simulink model "SiL_gram"  (R2025b)
settings: Solver=ode2  StartTime=0.0  StopTime=t_end  FixedStep=1/400  RelTol=1e-3
PreLoadFcn:
  | stepsize_sim = evalin('base', get_param(bdroot, 'FixedStep'));
undefined symbols (not defined in the file or in its folder): defaultConsts, defaultWP, DiscIntNeverNeededParam, dspblkCoreblockFVToolHelper, gcbh, navConsts, sensors, stepsize_ctrl
libraries: simulink x7, sharedutil x1, sharedtransform x1, aerolibanimutils x1
(part 2 of 3)

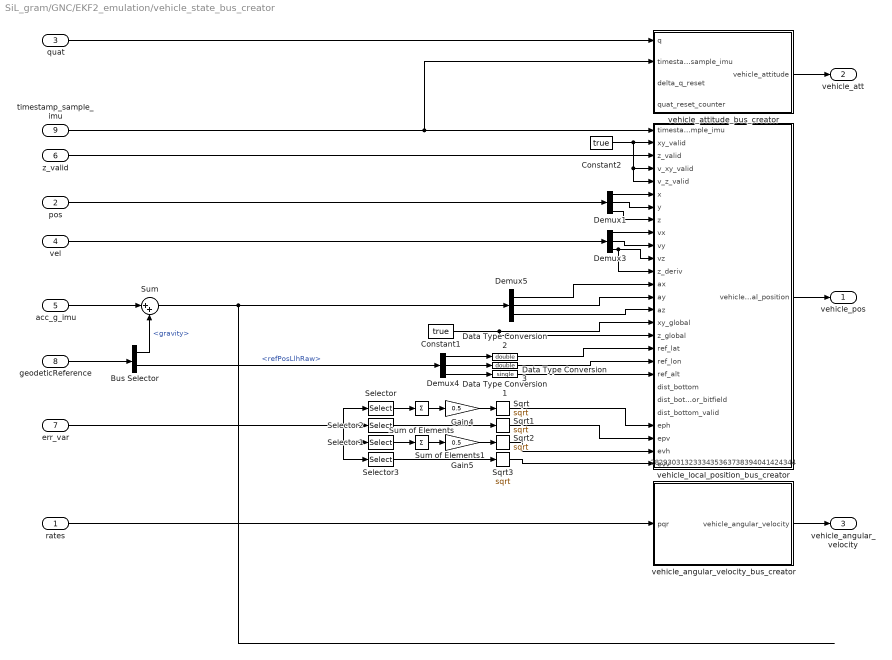
== system SiL_gram/GNC/EKF2_emulation/vehicle_state_bus_creator ==
  rates : Inport
  pos : Inport  Port=2  OutDataTypeStr=single  PortDimensions=3
  quat : Inport  Port=3
  vel : Inport  Port=4
  acc_g_imu : Inport  Port=5
  z_valid : Inport  Port=6  OutDataTypeStr=boolean
  err_var : Inport  Port=7
  geodeticReference : Inport  Port=8  OutDataTypeStr=Bus: ifr_geodeticReference
  timestamp_sample_imu : Inport  Port=9
  Bus Selector : BusSelector  OutputSignals=gravity,refPosLlhRaw
  Constant1 : Constant  Value=true  OutDataTypeStr=boolean
  Constant2 : Constant  Value=true  OutDataTypeStr=boolean
  Data Type Conversion1 : DataTypeConversion  OutDataTypeStr=double  SaturateOnIntegerOverflow=off  RndMeth=Floor
  Data Type Conversion2 : DataTypeConversion  OutDataTypeStr=double  SaturateOnIntegerOverflow=off  RndMeth=Floor
  Data Type Conversion3 : DataTypeConversion  OutDataTypeStr=single  SaturateOnIntegerOverflow=off  RndMeth=Floor
  Demux{1,3..5} (4 alike) : Demux  Outputs=3
  Gain4 : Gain  Gain=0.5  OutDataTypeStr=single
  Gain5 : Gain  Gain=0.5  OutDataTypeStr=single
  Selector : Selector  InputPortWidth=9  IndexOptions=Index vector (dialog)  Indices=[1 2]  OutputSizes=1
  Selector1 : Selector  InputPortWidth=9  IndexOptions=Index vector (dialog)  Indices=[4 5]  OutputSizes=1
  Selector2 : Selector  InputPortWidth=9  IndexOptions=Index vector (dialog)  Indices=3  OutputSizes=1
  Selector3 : Selector  InputPortWidth=9  IndexOptions=Index vector (dialog)  Indices=6  OutputSizes=1
  Sqrt{,1..3} (4 alike) : Sqrt
  Sum : Sum  Inputs=|++
  Sum of Elements : Sum  Inputs=+
  Sum of Elements1 : Sum  Inputs=+
  vehicle_angular_velocity_bus_creator : Subsystem
  vehicle_attitude_bus_creator : Subsystem
  vehicle_local_position_bus_creator : Subsystem
      settings: PortSchema="{\"entries\":[{\"content\":{\"sides\":[{\"content\":{\"connectorIds\":[\"In1\",\"In2\",\"In3\",\"In4\",\"In5\",\"In6\",\"In7\",\"In8\",\"In9\",\"In10\",\"In11\",\"In12\",\"In13\",\"In14\",\"In15\",\"In16\",\"In17\",\"In18\",\"In19\",\"In20\",\"In21\",\"In22\",\"In23\",\"In24\",\"In25\",\"In26\",\"In27\"]},\"type\":\"ConnectorPlacement.EquallySpacedRectSide\",\"uuid\":\"d7b85d5c-5599-4e88-82f1-b7fab1ef21b9\"},{\"content\":{\"connectorIds\":[\"Out1\"],\"side\":\"RIGHT\"},\"type\":\"ConnectorPlacement.EquallySpacedRectSide\",\"uuid\":\"699d4796-c4a5-400d-ae7f-d0fe809a1d5f\"},{\"content\":{\"side\":\"TOP\"},\"type\":\"ConnectorPlacement.EquallySpacedRectSide\",\"uuid\":\"a5a49804-595b-4b61-9074-ba74b998a229\"},{\"content\":{\"connectorIds\":[\"In28\",\"In29\",\"In30\",\"In31\",\"In32\",\"In33\",\"In34\",\"In35\",\"In36\",\"In37\",\"In38\",\"In39\",\"In40\",\"In41\",\"In42\",\"In43\",\"In44\"],\"side\":\"BOTTOM\"},\"type\":\"ConnectorPlacement.EquallySpacedRectSide\",\"uuid\":\"117ce955-faca-4d28-9193-e1fd103a05b2\"}]},\"type\":\"ConnectorPlacement.EquallySpacedConnector\",\"uuid\":\"4d71e442-d8d4-4e8b-a7eb-573f45a4a9ae\"}],\"packageUris\":[\"http://schema.mathworks.com/mf0/Connector/R2020b\"],\"version\":\"1.0\"}"
  vehicle_pos : Outport  OutDataTypeStr=Bus: vehicle_local_position_bus  VectorParamsAs1DForOutWhenUnconnected=off
  vehicle_att : Outport  Port=2  OutDataTypeStr=Bus: vehicle_attitude_bus  VectorParamsAs1DForOutWhenUnconnected=off
  vehicle_angular_velocity : Outport  Port=3  OutDataTypeStr=Bus: vehicle_angular_velocity_bus
  wires:
  rates/1 -> vehicle_angular_velocity_bus_creator/1(pqr)
  z_valid/1 -> vehicle_local_position_bus_creator/3(z_valid)
  Constant2/1 -> vehicle_local_position_bus_creator/4(v_xy_valid), vehicle_local_position_bus_creator/5(v_z_valid), vehicle_local_position_bus_creator/2(xy_valid)
  Demux5/3 -> vehicle_local_position_bus_creator/15(az)
  Data Type Conversion1/1 -> vehicle_local_position_bus_creator/19(ref_lon)
  Sqrt3/1 -> vehicle_local_position_bus_creator/27(evv)
  Sqrt2/1 -> vehicle_local_position_bus_creator/26(evh)
  vel/1 -> Demux3/1
  Demux4/3 -> Data Type Conversion3/1
  Sqrt1/1 -> vehicle_local_position_bus_creator/25(epv)
  Demux1/3 -> vehicle_local_position_bus_creator/8(z)
  Demux1/2 -> vehicle_local_position_bus_creator/7(y)
  Demux5/2 -> vehicle_local_position_bus_creator/14(ay)
  Constant1/1 -> vehicle_local_position_bus_creator/17(z_global), vehicle_local_position_bus_creator/16(xy_global)
  Demux1/1 -> vehicle_local_position_bus_creator/6(x)
  Data Type Conversion2/1 -> vehicle_local_position_bus_creator/18(ref_lat)
  Sqrt/1 -> vehicle_local_position_bus_creator/24(eph)
  Data Type Conversion3/1 -> vehicle_local_position_bus_creator/20(ref_alt)
  Demux3/3 -> vehicle_local_position_bus_creator/12(z_deriv), vehicle_local_position_bus_creator/11(vz)
  pos/1 -> Demux1/1
  Demux5/1 -> vehicle_local_position_bus_creator/13(ax)
  Demux3/1 -> vehicle_local_position_bus_creator/9(vx)
  Demux3/2 -> vehicle_local_position_bus_creator/10(vy)
  Selector1/1 -> Sum of Elements1/1
  Selector/1 -> Sum of Elements/1
  Selector3/1 -> Sqrt3/1
  Sum of Elements1/1 -> Gain5/1
  Sum of Elements/1 -> Gain4/1
  Selector2/1 -> Sqrt1/1
  err_var/1 -> Selector/1, Selector1/1, Selector3/1, Selector2/1
  Gain5/1 -> Sqrt2/1
  Gain4/1 -> Sqrt/1
  Sum/1 -> Demux5/1
  Bus Selector/2 -> Demux4/1  "<refPosLlhRaw>"
  Bus Selector/1 -> Sum/2  "<gravity>"
  geodeticReference/1 -> Bus Selector/1
  acc_g_imu/1 -> Sum/1
  quat/1 -> vehicle_attitude_bus_creator/1(q)
  timestamp_sample_imu/1 -> vehicle_attitude_bus_creator/2(timestamp_sample_imu), vehicle_local_position_bus_creator/1(timestamp_sample_imu)
  Demux4/2 -> Data Type Conversion1/1
  Demux4/1 -> Data Type Conversion2/1
  vehicle_local_position_bus_creator/1(vehicle_local_position) -> vehicle_pos/1
  vehicle_attitude_bus_creator/1(vehicle_attitude) -> vehicle_att/1
  vehicle_angular_velocity_bus_creator/1(vehicle_angular_velocity) -> vehicle_angular_velocity/1

== system SiL_gram/GNC/mavlink_receiver.cpp/  ==
  note: integration_timespan
      | ground_distance_m
  air : Inport  OutDataTypeStr=Bus: ifr_airdata
  Bus Creator1 : BusCreator  Inputs=21  OutDataTypeStr=Bus: optical_flow_bus
      settings: InheritFromInputs=off
  Bus Selector : BusSelector  OutputSignals=isValid,alpha_volt,beta_volt
  Constant1 : Constant  Value=zeros(3,1)
  Constant2 : Constant  Value=0  OutDataTypeStr=uint8
  Constant3 : Constant  Value=0  OutDataTypeStr=uint8
  Constant4 : Constant  Value=zeros(7,1)
  Constant5 : Constant  Value=0  OutDataTypeStr=single
  Constant6 : Constant  OutDataTypeStr=uint32
  Data Type Conversion{1..3,8..12} (8 alike) : DataTypeConversion  OutDataTypeStr=single  SaturateOnIntegerOverflow=off  RndMeth=Floor
  Data Type Conversion4 : DataTypeConversion  OutDataTypeStr=uint32  SaturateOnIntegerOverflow=off  RndMeth=Floor
  Data Type Conversion5 : DataTypeConversion  OutDataTypeStr=uint16  SaturateOnIntegerOverflow=off  RndMeth=Floor
  Data Type Conversion6 : DataTypeConversion  OutDataTypeStr=int16  SaturateOnIntegerOverflow=off  RndMeth=Floor
  Data Type Conversion7 : DataTypeConversion  OutDataTypeStr=uint8  SaturateOnIntegerOverflow=off  RndMeth=Floor
  Demux : Demux  Outputs=7
  Demux1 : Demux  Outputs=3
  opFlow : Outport  OutDataTypeStr=Bus: optical_flow_bus
  wires:
  Data Type Conversion8/1 -> Bus Creator1/14
  Constant1/1 -> Demux1/1
  Data Type Conversion2/1 -> Bus Creator1/6
  Data Type Conversion6/1 -> Bus Creator1/12
  Demux1/3 -> Data Type Conversion3/1
  Data Type Conversion3/1 -> Bus Creator1/7
  Demux/7 -> Data Type Conversion11/1
  Constant4/1 -> Demux/1
  Demux/4 -> Data Type Conversion7/1
  Data Type Conversion4/1 -> Bus Creator1/10
  Demux/5 -> Data Type Conversion8/1
  Demux/2 -> Data Type Conversion5/1
  Demux1/1 -> Data Type Conversion1/1
  Demux/6 -> Data Type Conversion9/1
  Constant5/1 -> Bus Creator1/8  "ground_distance_m"
  Bus Creator1/1 -> opFlow/1
  Constant3/1 -> Bus Creator1/2
  Data Type Conversion7/1 -> Bus Creator1/13
  Constant6/1 -> Bus Creator1/9  "integration_timespan"
  Data Type Conversion5/1 -> Bus Creator1/11
  Demux1/2 -> Data Type Conversion2/1
  Data Type Conversion11/1 -> Bus Creator1/16
  Demux/3 -> Data Type Conversion6/1
  Data Type Conversion9/1 -> Bus Creator1/15
  Data Type Conversion1/1 -> Bus Creator1/5
  Demux/1 -> Data Type Conversion4/1
  Data Type Conversion12/1 -> Bus Creator1/3
  air/1 -> Bus Selector/1
  Bus Selector/1 -> Bus Creator1/1  "<isValid>"
  Data Type Conversion10/1 -> Bus Creator1/4
  Bus Selector/3 -> Data Type Conversion10/1  "<beta_volt>"
  Bus Selector/2 -> Data Type Conversion12/1  "<alpha_volt>"
  Constant2/1 -> Bus Creator1/21, Bus Creator1/20, Bus Creator1/19, Bus Creator1/18, Bus Creator1/17

== system SiL_gram/GNC/mavlink_receiver.cpp/   ==
  Lidar : Inport  OutDataTypeStr=Bus: ifr_lidar
  Bus Creator1 : BusCreator  Inputs=31  OutDataTypeStr=Bus: distance_sensor_bus
      settings: InheritFromInputs=off
  Bus Selector : BusSelector  OutputSignals=isValid,distance
  Constant : Constant  Value=navConsts.lidarMinRange  OutDataTypeStr=single
  Constant1 : Constant  Value=navConsts.lidarMaxRange  OutDataTypeStr=single
  Constant11 : Constant  Value=zeros(4,1)  OutDataTypeStr=single
  Constant2 : Constant  Value=0  OutDataTypeStr=uint8
  Constant3 : Constant  OutDataTypeStr=uint8
  Constant4 : Constant  Value=0  OutDataTypeStr=int8
  Constant5 : Constant  OutDataTypeStr=uint8
  Constant6 : Constant  OutDataTypeStr=uint32
  Constant7 : Constant  Value=0  OutDataTypeStr=single
  Constant8 : Constant  Value=0  OutDataTypeStr=single
  Constant9 : Constant  Value=0  OutDataTypeStr=single
  lidar : Outport  OutDataTypeStr=Bus: distance_sensor_bus
  wires:
  Bus Creator1/1 -> lidar/1
  Lidar/1 -> Bus Selector/1
  Constant5/1 -> Bus Creator1/9  "MAV_DISTANCE_SENSOR_LASER"
  Constant/1 -> Bus Creator1/3
  Constant1/1 -> Bus Creator1/4
  Bus Selector/1 -> Bus Creator1/1  "<isValid>"
  Constant7/1 -> Bus Creator1/6
  Constant3/1 -> Bus Creator1/17  "ROTATION_DOWNWARD_FACING"
  Bus Selector/2 -> Bus Creator1/5  "<distance>"
  Constant4/1 -> Bus Creator1/7
  Constant6/1 -> Bus Creator1/2
  Constant8/1 -> Bus Creator1/13
  Constant9/1 -> Bus Creator1/14
  Constant11/1 -> Bus Creator1/15
  Constant2/1 -> Bus Creator1/12, Bus Creator1/11, Bus Creator1/10, Bus Creator1/8, Bus Creator1/31, Bus Creator1/30, Bus Creator1/29, Bus Creator1/28, Bus Creator1/27, Bus Creator1/26, Bus Creator1/25, Bus Creator1/24, Bus Creator1/23, Bus Creator1/22, Bus Creator1/21, Bus Creator1/20, Bus Creator1/19, Bus Creator1/18, Bus Creator1/16

== system SiL_gram/GNC/mavlink_receiver.cpp/    ==
  air : Inport  OutDataTypeStr=Bus: ifr_airdata
  Bus Creator1 : BusCreator  Inputs=6  OutDataTypeStr=Bus: airspeed_bus
      settings: InheritFromInputs=off
  Bus Selector : BusSelector  OutputSignals=isValid,V_a
  Cast To Double : DataTypeConversion  OutDataTypeStr=double  SaturateOnIntegerOverflow=off  RndMeth=Floor
  Constant1 : Constant  Value=0  OutDataTypeStr=single
  Constant2 : Constant  Value=0  OutDataTypeStr=single
  Constant3 : Constant  Value=0  OutDataTypeStr=single
  Data Type Conversion : DataTypeConversion  OutDataTypeStr=single  SaturateOnIntegerOverflow=off  RndMeth=Floor
  airdata : Outport  OutDataTypeStr=Bus: airspeed_bus
  wires:
  air/1 -> Bus Selector/1
  Data Type Conversion/1 -> Bus Creator1/3  "indicated_airspeed_m_s"
  Constant3/1 -> Bus Creator1/5  "air_temperature_celsius"
  Constant2/1 -> Bus Creator1/6  "confidence"
  Constant1/1 -> Bus Creator1/4  "true_airspeed_m_s"
  Bus Selector/1 -> Cast To Double/1, Bus Creator1/1  "<isValid>"
  Bus Creator1/1 -> airdata/1
  Bus Selector/2 -> Data Type Conversion/1  "<V_a>"
  Cast To Double/1 -> Bus Creator1/2  "true_airspeed_m_s"

== system SiL_gram/GNC/mavlink_receiver.cpp/ 1 ==
  air : Inport  OutDataTypeStr=Bus: ifr_airdata
  Bus Creator1 : BusCreator  Inputs=7  OutDataTypeStr=Bus: adc_report_bus
      settings: InheritFromInputs=off
  Bus Selector : BusSelector  OutputSignals=isValid,beta_volt,alpha_volt
  Constant : Constant  Value=[0,1,2,3,4,8,10,11,12,13,14,16]  OutDataTypeStr=int16
  Constant1 : Constant  Value=zeros(4,1)  OutDataTypeStr=single
  Constant2 : Constant  Value=zeros(5,1)  OutDataTypeStr=single
  Constant3 : Constant  Value=0  OutDataTypeStr=single
  Constant4 : Constant  OutDataTypeStr=uint32
  Constant5 : Constant  Value=zeros(12,1)  OutDataTypeStr=int32
  Constant6 : Constant  Value=0  OutDataTypeStr=uint32
  Constant7 : Constant  Value=0  OutDataTypeStr=single
  Mux : Mux  Inputs=5
  adcReport : Outport  OutDataTypeStr=Bus: adc_report_bus
  wires:
  Bus Selector/3 -> Mux/4  "<alpha_volt>"
  Bus Selector/2 -> Mux/2  "<beta_volt>"
  Bus Selector/1 -> Bus Creator1/1  "<isValid>"
  air/1 -> Bus Selector/1
  Bus Creator1/1 -> adcReport/1
  Constant/1 -> Bus Creator1/3
  Mux/1 -> Bus Creator1/4
  Constant1/1 -> Mux/1
  Constant2/1 -> Mux/3
  Constant3/1 -> Mux/5
  Constant4/1 -> Bus Creator1/2
  Constant5/1 -> Bus Creator1/5
  Constant6/1 -> Bus Creator1/6
  Constant7/1 -> Bus Creator1/7

== system SiL_gram/GNC/mavlink_receiver.cpp/Arming ==
  Bus Creator : BusCreator  Inputs=9  OutDataTypeStr=Bus: actuator_armed_bus
      settings: InheritFromInputs=off
  armed : Constant  OutDataTypeStr=boolean
  force_failsafe : Constant  Value=0  OutDataTypeStr=boolean
  in_esc_calibration_mode : Constant  Value=0  OutDataTypeStr=boolean
  is_valid : Constant  Value=0  OutDataTypeStr=boolean
  lockdown : Constant  Value=0  OutDataTypeStr=boolean
  manual_lockdown : Constant  OutDataTypeStr=boolean
  prearmed : Constant  Value=0  OutDataTypeStr=boolean
  ready_to_arm : Constant  Value=0  OutDataTypeStr=boolean
  soft_stop : Constant  Value=0  OutDataTypeStr=boolean
  Armed : Outport  OutDataTypeStr=Bus: actuator_armed_bus
  wires:
  Bus Creator/1 -> Armed/1
  soft_stop/1 -> Bus Creator/9
  in_esc_calibration_mode/1 -> Bus Creator/8
  ready_to_arm/1 -> Bus Creator/4
  is_valid/1 -> Bus Creator/1
  lockdown/1 -> Bus Creator/5
  manual_lockdown/1 -> Bus Creator/6
  armed/1 -> Bus Creator/2  "armed"
  prearmed/1 -> Bus Creator/3
  force_failsafe/1 -> Bus Creator/7

== system SiL_gram/GNC/mavlink_receiver.cpp/Baro ==
  note: [Pa]
  p_alt : Inport
  Bus Creator1 : BusCreator  Inputs=7  OutDataTypeStr=Bus: sensor_baro_bus
      settings: InheritFromInputs=off
  Bus Selector : BusSelector  OutputSignals=isValid,height
  Cast To Double : DataTypeConversion  OutDataTypeStr=double  SaturateOnIntegerOverflow=off  RndMeth=Floor
  Constant1 : Constant  Value=0  OutDataTypeStr=uint32
  Constant2 : Constant  OutDataTypeStr=uint32
  Constant3 : Constant  Value=0  OutDataTypeStr=double
  Constant4 : Constant  Value=0  OutDataTypeStr=uint8
  Data Type Conversion1 : DataTypeConversion  OutDataTypeStr=single  SaturateOnIntegerOverflow=off  RndMeth=Floor
  Data Type Conversion10 : DataTypeConversion  OutDataTypeStr=single  SaturateOnIntegerOverflow=off  RndMeth=Floor
  height2baro : MATLAB Function  TreatAsAtomicUnit=on
  baro : Outport  OutDataTypeStr=Bus: sensor_baro_bus
  wires:
  Constant4/1 -> Bus Creator1/7  "error_count"
  Constant2/1 -> Bus Creator1/3  "device_id"
  Constant3/1 -> Data Type Conversion1/1  "error_count"
  height2baro/1(pressure) -> Data Type Conversion10/1
  Bus Creator1/1 -> baro/1
  Data Type Conversion1/1 -> Bus Creator1/5  "temp"
  Bus Selector/2 -> height2baro/1(height)  "<height>"
  Bus Selector/1 -> Cast To Double/1, Bus Creator1/1  "<isValid>"
  Constant1/1 -> Bus Creator1/6  "error_count"
  Data Type Conversion10/1 -> Bus Creator1/4  "pressure"
  p_alt/1 -> Bus Selector/1
  Cast To Double/1 -> Bus Creator1/2  "true_airspeed_m_s"

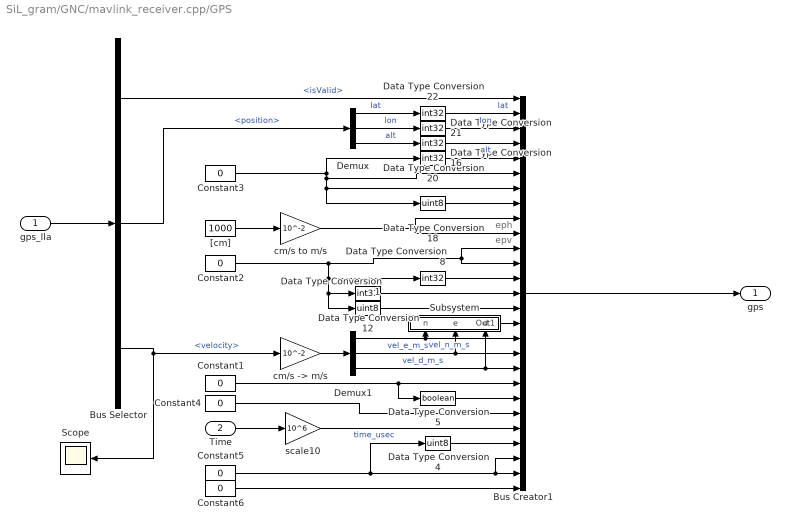
== system SiL_gram/GNC/mavlink_receiver.cpp/GPS ==
  note: eph
  note: epv
  gps_lla : Inport
  Time : Inport  Port=2
  Bus Creator1 : BusCreator  Inputs=27  OutDataTypeStr=Bus: vehicle_gps_position_bus
      settings: InheritFromInputs=off
  Bus Selector : BusSelector  OutputSignals=isValid,position,velocity
  Constant{1..3,5} (4 alike) : Constant  Value=0  OutDataTypeStr=single
  Constant4 : Constant  Value=0  OutDataTypeStr=int32
  Constant6 : Constant  Value=0  OutDataTypeStr=uint8
  Data Type Conversion1 : DataTypeConversion  OutDataTypeStr=uint8  SaturateOnIntegerOverflow=off  RndMeth=Floor
  Data Type Conversion{8,12,16,20..22} (6 alike) : DataTypeConversion  OutDataTypeStr=int32  SaturateOnIntegerOverflow=off  RndMeth=Floor
  Data Type Conversion18 : DataTypeConversion  OutDataTypeStr=uint8  SaturateOnIntegerOverflow=off  RndMeth=Floor
  Data Type Conversion4 : DataTypeConversion  OutDataTypeStr=uint8  SaturateOnIntegerOverflow=off  RndMeth=Floor
  Data Type Conversion5 : DataTypeConversion  OutDataTypeStr=boolean  SaturateOnIntegerOverflow=off  RndMeth=Floor
  Demux : Demux  Outputs=3
  Demux1 : Demux  Outputs=3
  Scope : Scope
      settings: ActiveDisplayYMinimum=-4879.31316  ActiveDisplayYMaximum=1977.92464
  Subsystem : Subsystem
      settings: PortSchema="{\"entries\":[{\"content\":{\"sides\":[{\"content\":{},\"type\":\"ConnectorPlacement.EquallySpacedRectSide\",\"uuid\":\"42608b9b-4e0b-4cd6-95a4-868653eebf85\"},{\"content\":{\"connectorIds\":[\"Out1\"],\"side\":\"RIGHT\"},\"type\":\"ConnectorPlacement.EquallySpacedRectSide\",\"uuid\":\"b8a148f6-1c9c-4225-91f9-202796ff464f\"},{\"content\":{\"side\":\"TOP\"},\"type\":\"ConnectorPlacement.EquallySpacedRectSide\",\"uuid\":\"0f80df07-b651-41b7-aa18-0093fc65c3ad\"},{\"content\":{\"connectorIds\":[\"In1\",\"In2\",\"In3\"],\"side\":\"BOTTOM\"},\"type\":\"ConnectorPlacement.EquallySpacedRectSide\",\"uuid\":\"f4234091-6e8c-4bc0-a362-f8928a822b26\"}]},\"type\":\"ConnectorPlacement.EquallySpacedConnector\",\"uuid\":\"4767cb59-0a97-4a99-80e8-760d373adfc4\"}],\"packageUris\":[\"http://schema.mathworks.com/mf0/Connector/R2020b\"],\"version\":\"1.0\"}"
  "[cm]" : Constant  Value=1000  OutDataTypeStr=single
  "cm/s -> m/s" : Gain  Gain=10^-2  OutDataTypeStr=single
  cm/s to m/s : Gain  Gain=10^-2  OutDataTypeStr=single
  scale10 : Gain  Gain=10^6  OutDataTypeStr=double
  gps : Outport  OutDataTypeStr=Bus: vehicle_gps_position_bus
  wires:
  Bus Selector/3 -> Scope/1, "cm/s -> m/s"/1  "<velocity>"
  Time/1 -> scale10/1
  Data Type Conversion22/1 -> Bus Creator1/2  "lat"
  Data Type Conversion21/1 -> Bus Creator1/3  "lon"
  Data Type Conversion20/1 -> Bus Creator1/4  "alt"
  Data Type Conversion18/1 -> Bus Creator1/8
  Data Type Conversion16/1 -> Bus Creator1/5
  Constant2/1 -> Bus Creator1/11, Bus Creator1/12, Data Type Conversion1/1, Data Type Conversion12/1, Data Type Conversion8/1
  Data Type Conversion12/1 -> Bus Creator1/14
  Data Type Conversion8/1 -> Bus Creator1/13
  Constant1/1 -> Bus Creator1/20, Data Type Conversion5/1
  Data Type Conversion5/1 -> Bus Creator1/21
  Data Type Conversion4/1 -> Bus Creator1/24
  Constant5/1 -> Data Type Conversion4/1, Bus Creator1/25, Bus Creator1/26
  scale10/1 -> Bus Creator1/23  "time_usec"
  Demux1/1 -> Subsystem/1(n), Bus Creator1/17  "vel_n_m_s"
  Demux1/2 -> Bus Creator1/18, Subsystem/2(e)  "vel_e_m_s"
  Demux1/3 -> Subsystem/3(d), Bus Creator1/19  "vel_d_m_s"
  Demux/3 -> Data Type Conversion20/1  "alt"
  Demux/2 -> Data Type Conversion21/1  "lon"
  Constant3/1 -> Data Type Conversion18/1, Bus Creator1/7, Bus Creator1/6, Data Type Conversion16/1
  Demux/1 -> Data Type Conversion22/1  "lat"
  Bus Creator1/1 -> gps/1
  Bus Selector/1 -> Bus Creator1/1  "<isValid>"
  gps_lla/1 -> Bus Selector/1
  Bus Selector/2 -> Demux/1  "<position>"
  "cm/s -> m/s"/1 -> Demux1/1
  "[cm]"/1 -> cm/s to m/s/1
  cm/s to m/s/1 -> Bus Creator1/9, Bus Creator1/10
  Constant4/1 -> Bus Creator1/22
  Data Type Conversion1/1 -> Bus Creator1/15
  Constant6/1 -> Bus Creator1/27
  Subsystem/1(Out1) -> Bus Creator1/16

== system SiL_gram/GNC/mavlink_receiver.cpp/InputRC ==
  note: 1 Thrust
      | 2 Aileron
      | 3 Elevator
      | 4 Rudder
      | 5 Tail surface right
      | 6 Tail surface left
      | 7 Mode switch
      | 8 Arming
      | 9 Safety
  note: [ Thrust ]
      | [ Aileron ]
      | [ Elevator ]
      | [ Rudder ]
      | [ NW ]
      | [ Mode ]
      | [ Safety ]
  note: Input from Gram RC:
      | 1 Thrust
      | 2 Aileron right
      | 3 Aileron left
      | 4 Flaperon right
      | 5 Flaperon left
      | 6 Elevator/Rudder right
      | 7 Elevator/Rudder left
      | 8 Gear
      | 9 Safety
      | 10 Arming
      | 11 Mode switch
      | 12 Elevator
      | 13 Rudder
  RC : Inport
  Bus Creator2 : BusCreator  Inputs=36  OutDataTypeStr=Bus: rc_channels_bus
      settings: InheritFromInputs=off
  Constant2 : Constant  Value=zeros(33,1)  OutDataTypeStr=uint8
  Constant3 : Constant  Value=zeros(12,1)  OutDataTypeStr=single
  Constant4 : Constant  Value=true
  Constant5 : Constant  Value=zeros(27,1)  OutDataTypeStr=int8
  Data Type Conversion : DataTypeConversion  OutDataTypeStr=single  SaturateOnIntegerOverflow=off  RndMeth=Floor
  Data Type Conversion1 : DataTypeConversion  OutDataTypeStr=double  SaturateOnIntegerOverflow=off  RndMeth=Floor
  Data Type Conversion2 : DataTypeConversion  OutDataTypeStr=boolean  SaturateOnIntegerOverflow=off  RndMeth=Floor
  Data Type Conversion4 : DataTypeConversion  OutDataTypeStr=uint8  SaturateOnIntegerOverflow=off  RndMeth=Floor
  Data Type Conversion6 : DataTypeConversion  OutDataTypeStr=single  SaturateOnIntegerOverflow=off  RndMeth=Floor
  Data Type Conversion7 : DataTypeConversion  OutDataTypeStr=uint8  SaturateOnIntegerOverflow=off  RndMeth=Floor
  Data Type Conversion8 : DataTypeConversion  OutDataTypeStr=uint32  SaturateOnIntegerOverflow=off  RndMeth=Floor
  Demux : Demux  Outputs=8
  Demux1 : Demux  Outputs=12
  Demux2 : Demux  Outputs=33
  Mux : Mux  Inputs=18
  Scope2 : Scope
      settings: ActiveDisplayYMinimum=-1.25  ActiveDisplayYMaximum=1.25
  Terminator1 : Terminator
  Terminator2 : Terminator
  rc_channels : Outport  OutDataTypeStr=Bus: rc_channels_bus
  wires:
  Demux/2 -> Mux/2
  Demux/6 -> Mux/7
  Demux/7 -> Mux/9
  Demux1/8 -> Mux/14
  Demux1/10 -> Mux/16
  Demux1/9 -> Mux/15
  RC/1 -> Data Type Conversion/1
  Data Type Conversion8/1 -> Bus Creator2/36
  Demux2/1 -> Bus Creator2/2
  Demux/5 -> Terminator1/1
  Demux1/11 -> Mux/17
  Data Type Conversion4/1 -> Bus Creator2/32
  Data Type Conversion1/1 -> Bus Creator2/30
  Demux2/32 -> Data Type Conversion2/1
  Demux2/29 -> Data Type Conversion1/1
  Demux2/9 -> Bus Creator2/10
  Constant5/1 -> Bus Creator2/33
  Demux2/26 -> Bus Creator2/27
  Demux2/17 -> Bus Creator2/18
  Demux2/10 -> Bus Creator2/11
  Data Type Conversion2/1 -> Bus Creator2/35
  Constant3/1 -> Demux1/1
  Demux2/31 -> Data Type Conversion7/1
  Constant2/1 -> Demux2/1
  Demux2/30 -> Data Type Conversion4/1
  Demux2/6 -> Bus Creator2/7
  Constant4/1 -> Bus Creator2/1
  Demux2/21 -> Bus Creator2/22
  Demux2/20 -> Bus Creator2/21
  Demux2/4 -> Bus Creator2/5
  Demux2/12 -> Bus Creator2/13
  Demux2/8 -> Bus Creator2/9
  Data Type Conversion6/1 -> Bus Creator2/31
  Demux2/22 -> Bus Creator2/23
  Demux1/12 -> Mux/18
  Demux2/23 -> Bus Creator2/24
  Demux2/24 -> Bus Creator2/25
  Demux2/19 -> Bus Creator2/20
  Demux2/13 -> Bus Creator2/14
  Demux2/2 -> Bus Creator2/3
  Mux/1 -> Data Type Conversion6/1, Scope2/1
  Demux2/33 -> Data Type Conversion8/1
  Demux2/11 -> Bus Creator2/12
  Demux2/3 -> Bus Creator2/4
  Demux2/25 -> Bus Creator2/26
  Demux2/16 -> Bus Creator2/17
  Demux2/7 -> Bus Creator2/8
  Demux2/14 -> Bus Creator2/15
  Data Type Conversion7/1 -> Bus Creator2/34
  Bus Creator2/1 -> rc_channels/1
  Demux2/15 -> Bus Creator2/16
  Demux/8 -> Terminator2/1
  Demux2/18 -> Bus Creator2/19
  Demux2/5 -> Bus Creator2/6
  Demux2/27 -> Bus Creator2/28
  Demux/1 -> Mux/1
  Demux1/6 -> Mux/12
  Data Type Conversion/1 -> Demux/1
  Demux2/28 -> Bus Creator2/29
  Demux1/2 -> Mux/6
  Demux/3 -> Mux/3
  Demux/4 -> Mux/4
  Demux1/7 -> Mux/13
  Demux1/1 -> Mux/5
  Demux1/3 -> Mux/8
  Demux1/4 -> Mux/10
  Demux1/5 -> Mux/11

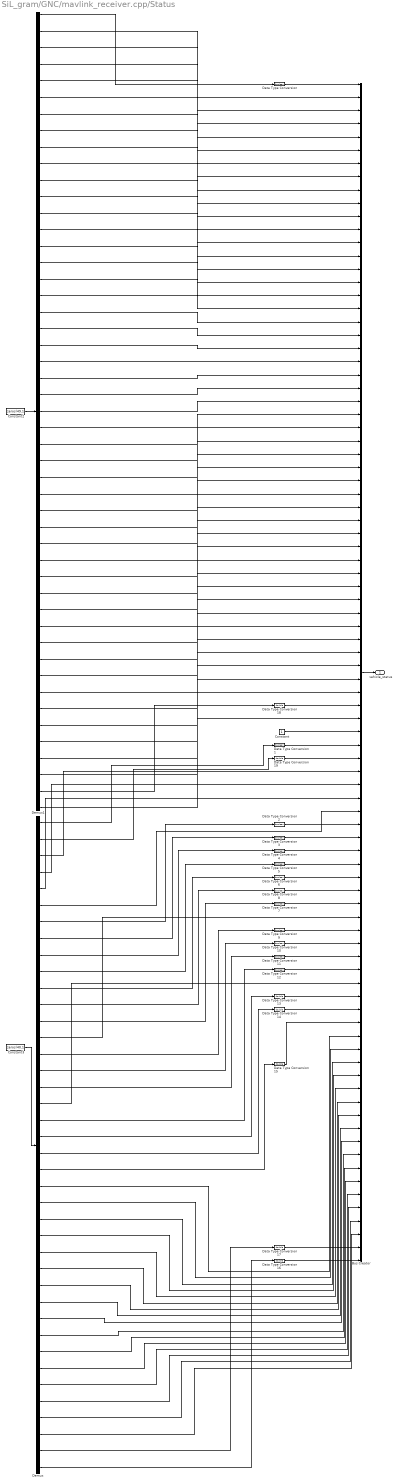
== system SiL_gram/GNC/mavlink_receiver.cpp/Status ==
  Bus Creator : BusCreator  Inputs=90  OutDataTypeStr=Bus: vehicle_status_bus
      settings: InheritFromInputs=off
  Constant : Constant  OutDataTypeStr=uint8
  Constant2 : Constant  Value=zeros(49,1)  OutDataTypeStr=uint8
  Constant3 : Constant  Value=zeros(40,1)  OutDataTypeStr=uint8
  Data Type Conversion{,1..12} (13 alike) : DataTypeConversion  OutDataTypeStr=boolean  SaturateOnIntegerOverflow=off  RndMeth=Floor
  Data Type Conversion{13..19} (7 alike) : DataTypeConversion  OutDataTypeStr=double  SaturateOnIntegerOverflow=off  RndMeth=Floor
  Demux : Demux  Outputs=40
  Demux1 : Demux  Outputs=49
  vehicle_status : Outport  OutDataTypeStr=Bus: vehicle_status_bus
  wires:
  Bus Creator/1 -> vehicle_status/1
  Data Type Conversion14/1 -> Bus Creator/71
  Data Type Conversion13/1 -> Bus Creator/70
  Data Type Conversion11/1 -> Bus Creator/67
  Data Type Conversion10/1 -> Bus Creator/66
  Data Type Conversion7/1 -> Bus Creator/63
  Data Type Conversion16/1 -> Bus Creator/90
  Data Type Conversion5/1 -> Bus Creator/60
  Data Type Conversion4/1 -> Bus Creator/59
  Data Type Conversion3/1 -> Bus Creator/58
  Data Type Conversion19/1 -> Bus Creator/52
  Data Type Conversion18/1 -> Bus Creator/48
  Data Type Conversion/1 -> Bus Creator/1
  Demux/39 -> Data Type Conversion17/1
  Demux/38 -> Bus Creator/88
  Demux/37 -> Bus Creator/87
  Data Type Conversion8/1 -> Bus Creator/62
  Demux/36 -> Bus Creator/86
  Demux/34 -> Bus Creator/84
  Demux/32 -> Bus Creator/82
  Demux/31 -> Bus Creator/81
  Demux/30 -> Bus Creator/80
  Data Type Conversion1/1 -> Bus Creator/51
  Demux/28 -> Bus Creator/78
  Demux/35 -> Bus Creator/85
  Demux/26 -> Bus Creator/76
  Demux/24 -> Bus Creator/74
  Demux/33 -> Bus Creator/83
  Demux/25 -> Bus Creator/75
  Demux/22 -> Data Type Conversion15/1
  Demux/21 -> Data Type Conversion14/1
  Demux/20 -> Data Type Conversion13/1
  Demux/16 -> Data Type Conversion10/1
  Demux/15 -> Data Type Conversion9/1
  Demux/14 -> Bus Creator/64
  Demux/12 -> Data Type Conversion8/1
  Demux/10 -> Data Type Conversion5/1
  Demux/9 -> Data Type Conversion4/1
  Demux1/24 -> Bus Creator/24
  Demux1/21 -> Bus Creator/21
  Demux1/20 -> Bus Creator/20
  Data Type Conversion12/1 -> Bus Creator/68
  Demux1/26 -> Bus Creator/26
  Demux1/25 -> Bus Creator/25
  Constant2/1 -> Demux1/1
  Demux1/41 -> Bus Creator/41
  Demux1/45 -> Bus Creator/45
  Demux1/18 -> Bus Creator/18
  Demux1/42 -> Bus Creator/42
  Demux1/39 -> Bus Creator/39
  Demux1/12 -> Bus Creator/12
  Demux1/15 -> Bus Creator/15
  Demux1/27 -> Bus Creator/27
  Constant/1 -> Bus Creator/50
  Demux/1 -> Data Type Conversion1/1
  Demux/18 -> Bus Creator/69
  Demux1/2 -> Bus Creator/2
  Demux1/7 -> Bus Creator/7
  Demux/3 -> Bus Creator/53
  Demux1/14 -> Bus Creator/14
  Demux1/46 -> Bus Creator/46
  Constant3/1 -> Demux/1
  Demux/4 -> Bus Creator/54
  Demux1/43 -> Bus Creator/43
  Demux/40 -> Data Type Conversion16/1
  Demux/11 -> Data Type Conversion6/1
  Demux1/22 -> Bus Creator/22
  Demux1/13 -> Bus Creator/13
  Demux1/4 -> Bus Creator/4
  Demux1/3 -> Bus Creator/3
  Demux1/6 -> Bus Creator/6
  Demux1/32 -> Bus Creator/32
  Demux1/10 -> Bus Creator/10
  Data Type Conversion6/1 -> Bus Creator/61
  Data Type Conversion2/1 -> Bus Creator/57
  Demux1/19 -> Bus Creator/19
  Demux/8 -> Data Type Conversion3/1
  Demux1/30 -> Bus Creator/30
  Demux1/23 -> Bus Creator/23
  Demux/13 -> Data Type Conversion7/1
  Demux1/49 -> Bus Creator/49
  Demux1/5 -> Bus Creator/5
  Demux1/9 -> Bus Creator/9
  Data Type Conversion9/1 -> Bus Creator/65
  Demux1/11 -> Bus Creator/11
  Demux1/17 -> Bus Creator/17
  Demux1/29 -> Bus Creator/29
  Demux/23 -> Bus Creator/73
  Demux1/28 -> Bus Creator/28
  Demux1/31 -> Bus Creator/31
  Demux1/33 -> Bus Creator/33
  Data Type Conversion17/1 -> Bus Creator/89
  Demux/19 -> Data Type Conversion12/1
  Demux1/34 -> Bus Creator/34
  Demux1/35 -> Bus Creator/35
  Demux/29 -> Bus Creator/79
  Demux1/37 -> Bus Creator/37
  Demux1/16 -> Bus Creator/16
  Demux1/40 -> Bus Creator/40
  Demux1/8 -> Bus Creator/8
  Demux1/44 -> Bus Creator/44
  Demux1/38 -> Bus Creator/38
  Demux1/47 -> Bus Creator/47
  Demux/17 -> Data Type Conversion11/1
  Demux1/1 -> Data Type Conversion/1
  Demux1/36 -> Bus Creator/36
  Demux1/48 -> Data Type Conversion18/1
  Data Type Conversion15/1 -> Bus Creator/72
  Demux/2 -> Data Type Conversion19/1
  Demux/5 -> Bus Creator/55
  Demux/27 -> Bus Creator/77
  Demux/6 -> Bus Creator/56
  Demux/7 -> Data Type Conversion2/1

== system SiL_gram/GNC/mavlink_receiver.cpp/Subsystem ==
  rate : Inport
  Bus Creator2 : BusCreator  Inputs=10  OutDataTypeStr=Bus: sensor_gyro_bus
      settings: InheritFromInputs=off
  Constant1 : Constant  Value=true  OutDataTypeStr=double
  Constant2 : Constant  Value=0  OutDataTypeStr=double
  Constant3 : Constant  Value=0  OutDataTypeStr=double
  Constant4 : Constant  Value=0  OutDataTypeStr=double
  Constant5 : Constant  Value=true  OutDataTypeStr=boolean
  Constant6 : Constant  OutDataTypeStr=uint32
  Constant7 : Constant  Value=0  OutDataTypeStr=uint32
  Data Type Conversion1 : DataTypeConversion  OutDataTypeStr=single  SaturateOnIntegerOverflow=off  RndMeth=Floor
  Data Type Conversion2 : DataTypeConversion  OutDataTypeStr=uint8  SaturateOnIntegerOverflow=off  RndMeth=Floor
  Data Type Conversion3 : DataTypeConversion  OutDataTypeStr=uint8  SaturateOnIntegerOverflow=off  RndMeth=Floor
  Data Type Conversion6 : DataTypeConversion  OutDataTypeStr=single  SaturateOnIntegerOverflow=off  RndMeth=Floor
  Demux3 : Demux  Outputs=3
  Gyro : Outport  OutDataTypeStr=Bus: sensor_gyro_bus
  wires:
  Bus Creator2/1 -> Gyro/1
  Data Type Conversion3/1 -> Bus Creator2/10
  rate/1 -> Data Type Conversion6/1
  Constant6/1 -> Bus Creator2/3  "device_id"
  Data Type Conversion6/1 -> Demux3/1
  Data Type Conversion1/1 -> Bus Creator2/7
  Data Type Conversion2/1 -> Bus Creator2/9
  Constant2/1 -> Data Type Conversion1/1  "error_count"
  Demux3/3 -> Bus Creator2/6  "z"
  Constant3/1 -> Data Type Conversion2/1  "error_count"
  Demux3/1 -> Bus Creator2/4  "x"
  Constant4/1 -> Data Type Conversion3/1  "error_count"
  Constant7/1 -> Bus Creator2/8  "error_count"
  Constant5/1 -> Bus Creator2/1  "is_valid"
  Constant1/1 -> Bus Creator2/2  "is_valid"
  Demux3/2 -> Bus Creator2/5  "y"

== system SiL_gram/GNC/mavlink_receiver.cpp/Subsystem1 ==
  <accel> : Inport
  Bus Creator1 : BusCreator  Inputs=11  OutDataTypeStr=Bus: sensor_accel_bus
      settings: InheritFromInputs=off
  Constant1 : Constant  Value=true  OutDataTypeStr=boolean
  Constant2 : Constant  OutDataTypeStr=uint32
  Constant3 : Constant  Value=0  OutDataTypeStr=double
  Constant4 : Constant  Value=zeros(3,1)
  Constant5 : Constant  Value=true  OutDataTypeStr=double
  Constant6 : Constant  Value=0  OutDataTypeStr=uint32
  Constant8 : Constant  Value=0  OutDataTypeStr=double
  Constant9 : Constant  Value=0  OutDataTypeStr=double
  Data Type Conversion11 : DataTypeConversion  OutDataTypeStr=single  SaturateOnIntegerOverflow=off  RndMeth=Floor
  Data Type Conversion12 : DataTypeConversion  OutDataTypeStr=uint8  SaturateOnIntegerOverflow=off  RndMeth=Floor
  Data Type Conversion13 : DataTypeConversion  OutDataTypeStr=uint8  SaturateOnIntegerOverflow=off  RndMeth=Floor
  Data Type Conversion14 : DataTypeConversion  OutDataTypeStr=uint8  SaturateOnIntegerOverflow=off  RndMeth=Floor
  Data Type Conversion3 : DataTypeConversion  OutDataTypeStr=single  SaturateOnIntegerOverflow=off  RndMeth=Floor
  Demux1 : Demux  Outputs=3
  accel : Outport  OutDataTypeStr=Bus: sensor_accel_bus
  wires:
  Data Type Conversion14/1 -> Bus Creator1/11
  Data Type Conversion13/1 -> Bus Creator1/10
  Data Type Conversion12/1 -> Bus Creator1/9
  <accel>/1 -> Data Type Conversion3/1
  Demux1/3 -> Bus Creator1/6  "z"
  Data Type Conversion3/1 -> Demux1/1
  Constant3/1 -> Data Type Conversion11/1  "error_count"
  Constant2/1 -> Bus Creator1/3  "device_id"
  Constant4/1 -> Data Type Conversion12/1  "error_count"
  Demux1/2 -> Bus Creator1/5  "y"
  Bus Creator1/1 -> accel/1
  Constant8/1 -> Data Type Conversion13/1  "error_count"
  Constant1/1 -> Bus Creator1/1  "is_valid"
  Constant9/1 -> Data Type Conversion14/1  "error_count"
  Constant6/1 -> Bus Creator1/8  "error_count"
  Constant5/1 -> Bus Creator1/2  "is_valid"
  Demux1/1 -> Bus Creator1/4  "x"
  Data Type Conversion11/1 -> Bus Creator1/7

== system SiL_gram/GNC/mavlink_receiver.cpp/Waypoints ==
  Bus Creator : BusCreator  Inputs=5  OutDataTypeStr=Bus: waypoint_list_bus
      settings: InheritFromInputs=off
  Bus Selector : BusSelector  OutputSignals=is_valid,lat,lon,alt,count
  Geodetic Reference : MATLAB Function  TreatAsAtomicUnit=on
  MATLAB Function2 : MATLAB Function  TreatAsAtomicUnit=on
  Manual Switch : ManualSwitch
  switch WPs : Subsystem
  WP_lla : Outport  OutDataTypeStr=Bus: waypoint_list_bus
  wires:
  Geodetic Reference/1(refPos) -> MATLAB Function2/1(refPos)
  switch WPs/1(original) -> Manual Switch/1
  switch WPs/2(modified) -> Manual Switch/2
  Manual Switch/1 -> MATLAB Function2/3(flightplan)
  Geodetic Reference/2(llh2ned) -> MATLAB Function2/2(llh2ned)
  MATLAB Function2/1(wp_lla) -> Bus Selector/1
  Bus Creator/1 -> WP_lla/1
  Bus Selector/1 -> Bus Creator/1  "<is_valid>"
  Bus Selector/2 -> Bus Creator/2  "<lat>"
  Bus Selector/4 -> Bus Creator/4  "<alt>"
  Bus Selector/3 -> Bus Creator/3  "<lon>"
  Bus Selector/5 -> Bus Creator/5  "<count>"

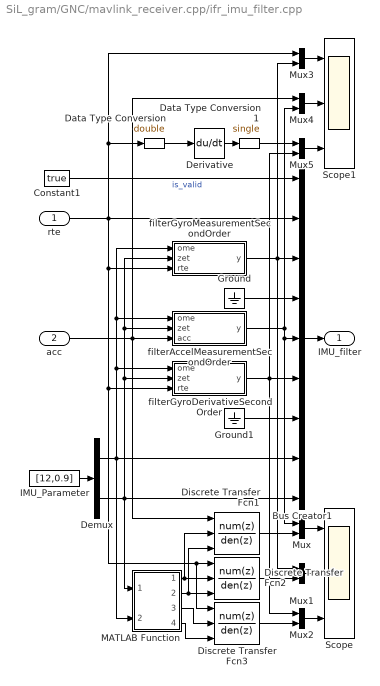
== system SiL_gram/GNC/mavlink_receiver.cpp/ifr_imu_filter.cpp ==
  rte : Inport
  acc : Inport  Port=2
  Bus Creator1 : BusCreator  Inputs=9  OutDataTypeStr=Bus: ifr_imu_filtered_bus
      settings: InheritFromInputs=off
  Constant1 : Constant  Value=true  OutDataTypeStr=boolean
  Data Type Conversion : DataTypeConversion  OutDataTypeStr=double  SaturateOnIntegerOverflow=off  RndMeth=Floor
  Data Type Conversion1 : DataTypeConversion  OutDataTypeStr=single  SaturateOnIntegerOverflow=off  RndMeth=Floor
  Demux : Demux  Outputs=2
  Derivative : Derivative
  Discrete Transfer Fcn1 : DiscreteTransferFcn  NumeratorSource=Input port  DenominatorSource=Input port  a0EqualsOne=on
      settings: InputPortMap=u0,p1,p3
  Discrete Transfer Fcn2 : DiscreteTransferFcn  NumeratorSource=Input port  DenominatorSource=Input port  a0EqualsOne=on
      settings: InputPortMap=u0,p1,p3
  Discrete Transfer Fcn3 : DiscreteTransferFcn  NumeratorSource=Input port  DenominatorSource=Input port  a0EqualsOne=on
      settings: InputPortMap=u0,p1,p3
  Ground : Ground
  Ground1 : Ground
  IMU_Parameter : Constant  Value=[12,0.9]  OutDataTypeStr=single
  MATLAB Function : MATLAB Function  TreatAsAtomicUnit=on
  Mux{,1..5} (6 alike) : Mux  Inputs=2
  Scope : Scope  NumInputPorts=3
      settings: ActiveDisplayYMinimum=-0.010298976601916364  ActiveDisplayYMaximum=0.075779346327180974  DataLoggingVariableName=ScopeData4
  Scope1 : Scope  NumInputPorts=3
      settings: ActiveDisplayYMinimum=-1.432850182056427  ActiveDisplayYMaximum=1.7771502137184143
  filterAccelMeasurementSecondOrder : MATLAB Function  TreatAsAtomicUnit=on
  filterGyroDerivativeSecondOrder : MATLAB Function  TreatAsAtomicUnit=on
  filterGyroMeasurementSecondOrder : MATLAB Function  TreatAsAtomicUnit=on
  IMU_filter : Outport  OutDataTypeStr=Bus: ifr_imu_filtered_bus
  wires:
  Constant1/1 -> Bus Creator1/1  "is_valid"
  Bus Creator1/1 -> IMU_filter/1
  IMU_Parameter/1 -> Demux/1
  Demux/1 -> filterGyroDerivativeSecondOrder/1(ome), filterAccelMeasurementSecondOrder/1(ome), filterGyroMeasurementSecondOrder/1(ome), MATLAB Function/2(omega), Bus Creator1/8
  Demux/2 -> filterGyroDerivativeSecondOrder/2(zet), filterAccelMeasurementSecondOrder/2(zet), filterGyroMeasurementSecondOrder/2(zet), MATLAB Function/1(zeta), Bus Creator1/9
  acc/1 -> Discrete Transfer Fcn1/1, Mux4/1, filterAccelMeasurementSecondOrder/3(acc)
  rte/1 -> Discrete Transfer Fcn3/1, Discrete Transfer Fcn2/1, filterGyroDerivativeSecondOrder/3(rte), filterGyroMeasurementSecondOrder/3(rte), Mux3/1, Data Type Conversion/1, Bus Creator1/2
  filterGyroMeasurementSecondOrder/1(y) -> Mux1/1, Mux3/2, Bus Creator1/3
  Ground/1 -> Bus Creator1/4
  filterAccelMeasurementSecondOrder/1(y) -> Mux/1, Bus Creator1/5, Mux4/2
  filterGyroDerivativeSecondOrder/1(y) -> Mux2/1, Mux5/2, Bus Creator1/6
  Ground1/1 -> Bus Creator1/7
  MATLAB Function/4(diff_den) -> Discrete Transfer Fcn3/3
  MATLAB Function/3(diff_num) -> Discrete Transfer Fcn3/2
  MATLAB Function/2(filt_den) -> Discrete Transfer Fcn1/3, Discrete Transfer Fcn2/3
  MATLAB Function/1(filt_num) -> Discrete Transfer Fcn2/2, Discrete Transfer Fcn1/2
  Discrete Transfer Fcn1/1 -> Mux/2
  Discrete Transfer Fcn2/1 -> Mux1/2
  Discrete Transfer Fcn3/1 -> Mux2/2
  Mux1/1 -> Scope/2
  Mux2/1 -> Scope/3
  Mux/1 -> Scope/1
  Mux5/1 -> Scope1/3
  Mux4/1 -> Scope1/2
  Derivative/1 -> Data Type Conversion1/1
  Mux3/1 -> Scope1/1
  Data Type Conversion/1 -> Derivative/1
  Data Type Conversion1/1 -> Mux5/1

== system SiL_gram/Remote_Control/Subsystem3/Variant 1 ==
  note: Aileron
      |
      |
      |
      | Elevator
      |
      |
      |
      | Thrust
      |
      |
      |
      | Rudder/TW
      |
      |
      |
      | Unused
  Constant11 : Constant  Value=0
  Constant12 : Constant  Value=0
  Constant13 : Constant  Value=0
  Mux3 : Mux  Inputs=5
  Ramp : simulink/Sources/Ramp  slope=0.5  start=4  InitialOutput=0
  Ramp1 : simulink/Sources/Ramp  slope=-0.5  start=2  InitialOutput=1
  Saturation : Saturate  UpperLimit=0.15  LowerLimit=0
  Saturation1 : Saturate  UpperLimit=1  LowerLimit=0
  Scope1 : Scope
      settings: ActiveDisplayYMinimum=-0.125  ActiveDisplayYMaximum=1.125  DataLoggingVariableName=ScopeData3
  Axes : Outport
  wires:
  Ramp1/1 -> Saturation1/1
  Constant12/1 -> Mux3/5
  Saturation1/1 -> Mux3/3
  Ramp/1 -> Saturation/1
  Saturation/1 -> Mux3/4
  Constant13/1 -> Mux3/1
  Constant11/1 -> Mux3/2
  Mux3/1 -> Axes/1, Scope1/1

== system SiL_gram/Remote_Control/Subsystem3/Variant 2 ==
  note: Aileron
      |
      |
      |
      | Elevator
      |
      |
      |
      | Thrust
      |
      |
      |
      | Rudder/TW
      |
      |
      |
      | Unused
  Constant{1,11..13} (4 alike) : Constant  Value=0
  Mux3 : Mux  Inputs=5
  Ramp1 : simulink/Sources/Ramp  slope=-0.5  start=0  InitialOutput=1
  Saturation1 : Saturate  UpperLimit=1  LowerLimit=-1
  Scope1 : Scope
      settings: ActiveDisplayYMinimum=-1.25  ActiveDisplayYMaximum=1.25  DataLoggingVariableName=ScopeData2
  Step : Step  Time=4  Before=1  After=-1  SampleTime=0
  Terminator : Terminator
  Axes : Outport
  wires:
  Constant11/1 -> Mux3/2
  Constant13/1 -> Mux3/1
  Constant1/1 -> Mux3/4
  Saturation1/1 -> Mux3/3
  Constant12/1 -> Mux3/5
  Step/1 -> Saturation1/1
  Mux3/1 -> Axes/1, Scope1/1
  Ramp1/1 -> Terminator/1

== system SiL_gram/Remote_Control/Subsystem3/Variant 3 ==
  Constant1 : Constant  Value=[0 0 1 0 0]'
  Axes : Outport
  wires:
  Constant1/1 -> Axes/1

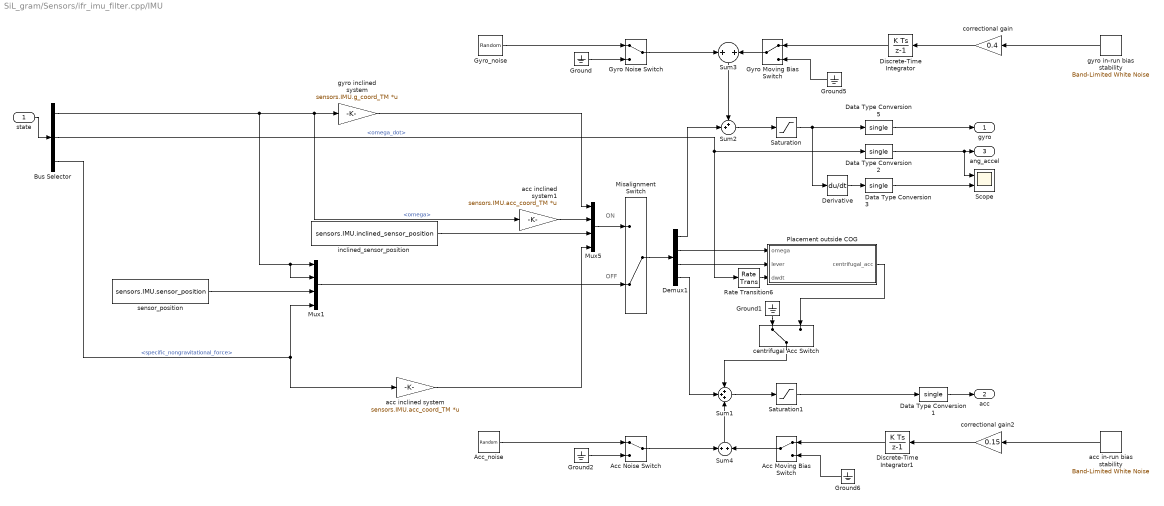
== system SiL_gram/Sensors/ifr_imu_filter.cpp/IMU ==
  note: ON
  note: OFF
  state : Inport  OutDataTypeStr=Bus: fmBus
  Acc Moving Bias Switch : ManualSwitch
  Acc Noise Switch : ManualSwitch
  Acc_noise : RandomNumber  Mean=sensors.IMU.acc_initial_bias  Variance=sensors.IMU.acc_noise^2*[1 1 1]  Seed=[6 7 8]  SampleTime=sensors.IMU.timestep
  Bus Selector : BusSelector  OutputSignals=rigidbodyBus.omega,utilityBus.omega_dot,utilityBus.specific_nongravitational_force
  Data Type Conversion{1..3,5} (4 alike) : DataTypeConversion  OutDataTypeStr=single  SaturateOnIntegerOverflow=off  RndMeth=Floor
  Demux1 : Demux
  Derivative : Derivative
  Discrete-Time Integrator : DiscreteIntegrator  SampleTime=-1  ICPrevOutput=DiscIntNeverNeededParam  ICPrevScaledInput=DiscIntNeverNeededParam
  Discrete-Time Integrator1 : DiscreteIntegrator  SampleTime=-1  ICPrevOutput=DiscIntNeverNeededParam  ICPrevScaledInput=DiscIntNeverNeededParam
  Ground{,1..2,5..6} (5 alike) : Ground
  Gyro Moving Bias Switch : ManualSwitch
  Gyro Noise Switch : ManualSwitch
  Gyro_noise : RandomNumber  Mean=sensors.IMU.g_initial_bias  Variance=sensors.IMU.g_noise^2*[1 1 1]  Seed=[0 1 2]  SampleTime=sensors.IMU.timestep
  Misalignment Switch : ManualSwitch  CurrentSetting=0
  Mux1 : Mux
  Mux5 : Mux
  Placement outside COG : MATLAB Function  TreatAsAtomicUnit=on
  Rate Transition6 : RateTransition  OutPortSampleTime=stepsize_sens
  Saturation : Saturate  UpperLimit=sensors.IMU.g_range  LowerLimit=-sensors.IMU.g_range
  Saturation1 : Saturate  UpperLimit=sensors.IMU.acc_range  LowerLimit=-sensors.IMU.acc_range
  Scope : Scope  NumInputPorts=2
      settings: ActiveDisplayYMinimum=-153.87794303894043  ActiveDisplayYMaximum=89.505979537963867  DataLoggingVariableName=ScopeData8
  Sum1 : Sum  Inputs=+++
  Sum2 : Sum  Inputs=++|
  Sum3 : Sum
  Sum4 : Sum
  acc in-run bias stability : simulink/Sources/Band-Limited White Noise  Cov=sensors.IMU.acc_inrun_bias^2*[1 1 1]  Ts=sensors.IMU.timestep  seed=[40 31 56]
  acc inclined system : Gain  Gain=sensors.IMU.acc_coord_TM  Multiplication=Matrix(K*u)
  acc inclined system1 : Gain  Gain=sensors.IMU.acc_coord_TM  Multiplication=Matrix(K*u)
  centrifugal Acc Switch : ManualSwitch
  correctional gain : Gain  Gain=0.4
  correctional gain2 : Gain  Gain=0.15
  gyro in-run bias stability : simulink/Sources/Band-Limited White Noise  Cov=sensors.IMU.g_inrun_bias^2*[1 1 1]  Ts=sensors.IMU.timestep  seed=[21 30 27]
  gyro inclined system : Gain  Gain=sensors.IMU.g_coord_TM  Multiplication=Matrix(K*u)
  inclined_sensor_position : Constant  Value=sensors.IMU.inclined_sensor_position
  sensor_position : Constant  Value=sensors.IMU.sensor_position
  gyro : Outport
  acc : Outport  Port=2
  ang_accel : Outport  Port=3
  wires:
  state/1 -> Bus Selector/1
  Demux1/4 -> Sum1/2
  Ground5/1 -> Gyro Moving Bias Switch/2
  Saturation1/1 -> Data Type Conversion1/1
  Sum3/1 -> Sum2/1
  gyro inclined system/1 -> Mux5/1
  Ground/1 -> Gyro Noise Switch/2
  Ground6/1 -> Acc Moving Bias Switch/2
  Mux5/1 -> Misalignment Switch/1
  Mux1/1 -> Misalignment Switch/2
  Gyro_noise/1 -> Gyro Noise Switch/1
  correctional gain/1 -> Discrete-Time Integrator/1
  Demux1/3 -> Placement outside COG/2(lever)
  Sum2/1 -> Saturation/1
  Acc Moving Bias Switch/1 -> Sum4/2
  Acc Noise Switch/1 -> Sum4/1
  Placement outside COG/1(centrifugal_acc) -> centrifugal Acc Switch/2
  Bus Selector/2 -> Rate Transition6/1, Data Type Conversion2/1  "<omega_dot>"
  Data Type Conversion1/1 -> acc/1
  inclined_sensor_position/1 -> Mux5/3
  gyro in-run bias stability/1 -> correctional gain/1
  Misalignment Switch/1 -> Demux1/1
  Data Type Conversion5/1 -> gyro/1
  centrifugal Acc Switch/1 -> Sum1/1
  Discrete-Time Integrator1/1 -> Acc Moving Bias Switch/1
  Demux1/1 -> Sum2/2
  Ground1/1 -> centrifugal Acc Switch/1
  Bus Selector/3 -> acc inclined system/1, Mux1/4  "<specific_nongravitational_force>"
  Rate Transition6/1 -> Placement outside COG/3(dwdt)
  Demux1/2 -> Placement outside COG/1(omega)
  Ground2/1 -> Acc Noise Switch/2
  acc inclined system1/1 -> Mux5/2
  Bus Selector/1 -> Mux1/1, Mux1/2, gyro inclined system/1, acc inclined system1/1  "<omega>"
  Saturation/1 -> Data Type Conversion5/1, Derivative/1
  correctional gain2/1 -> Discrete-Time Integrator1/1
  acc inclined system/1 -> Mux5/4
  acc in-run bias stability/1 -> correctional gain2/1
  Gyro Noise Switch/1 -> Sum3/1
  Sum1/1 -> Saturation1/1
  Discrete-Time Integrator/1 -> Gyro Moving Bias Switch/1
  Acc_noise/1 -> Acc Noise Switch/1
  Sum4/1 -> Sum1/3
  Gyro Moving Bias Switch/1 -> Sum3/2
  sensor_position/1 -> Mux1/3
  Derivative/1 -> Data Type Conversion3/1
  Data Type Conversion2/1 -> Scope/1, ang_accel/1
  Data Type Conversion3/1 -> Scope/2

== system SiL_gram/GNC/EKF2_emulation/vehicle_state_bus_creator/vehicle_angular_velocity_bus_creator ==
  pqr : Inport  OutDataTypeStr=single  PortDimensions=3
  Bus Creator1 : BusCreator  Inputs=3  OutDataTypeStr=Bus: vehicle_angular_velocity_bus
      settings: InheritFromInputs=off
  Ground : Ground
  is_valid : Constant  Value=true  OutDataTypeStr=boolean
  vehicle_angular_velocity : Outport  OutDataTypeStr=Bus: vehicle_angular_velocity_bus
  wires:
  pqr/1 -> Bus Creator1/3
  Ground/1 -> Bus Creator1/2
  is_valid/1 -> Bus Creator1/1
  Bus Creator1/1 -> vehicle_angular_velocity/1

== system SiL_gram/GNC/EKF2_emulation/vehicle_state_bus_creator/vehicle_attitude_bus_creator ==
  q : Inport  OutDataTypeStr=single  PortDimensions=4
  timestamp_sample_imu : Inport  Port=2
  delta_q_reset : Inport  Port=3  OutDataTypeStr=single  PortDimensions=4
  quat_reset_counter : Inport  Port=4  OutDataTypeStr=uint8  PortDimensions=1
  Bus Creator : BusCreator  Inputs=5  OutDataTypeStr=Bus: vehicle_attitude_bus
      settings: InheritFromInputs=off
  is_valid : Constant  Value=true  OutDataTypeStr=boolean
  vehicle_attitude : Outport  OutDataTypeStr=Bus: vehicle_attitude_bus  VectorParamsAs1DForOutWhenUnconnected=off
  wires:
  is_valid/1 -> Bus Creator/1
  timestamp_sample_imu/1 -> Bus Creator/2
  q/1 -> Bus Creator/3
  delta_q_reset/1 -> Bus Creator/4
  quat_reset_counter/1 -> Bus Creator/5
  Bus Creator/1 -> vehicle_attitude/1
